simulink model "VehicleDynamics2011"  (Simulink 7.8)
settings: Solver=ode3  StartTime=0.0  StopTime=130  RelTol=1e-3
values from neighbouring files (symbols this model uses):
  b = 100    [parameters.m]
  L1 = 1.6    [parameters.m]
  m = 2000    [parameters.m]
undefined symbols (not defined in the file or in its folder): DiscIntNeverNeededParam
libraries: simulink x2
settings Model: Creator=jmapatel  LastModifiedBy=minzhe
settings OptimizationCC: InitFltsAndDblsToZero=on
settings DebuggingCC: SaveWithParameterizedLinksMsg=none  SignalResolutionControl=TryResolveAllWithWarning  MultiTaskDSMMsg=warning  MultiTaskCondExecSysMsg=none  FcnCallInpInsideContextMsg=Use local settings
settings CodeAppCC: CustomSymbolStrType=$N$R$M_T
settings GRTTargetCC: TargetFcnLib=ansi_tfl_tmw.mat  TargetFunctionLibrary=C89/C90 (ANSI)

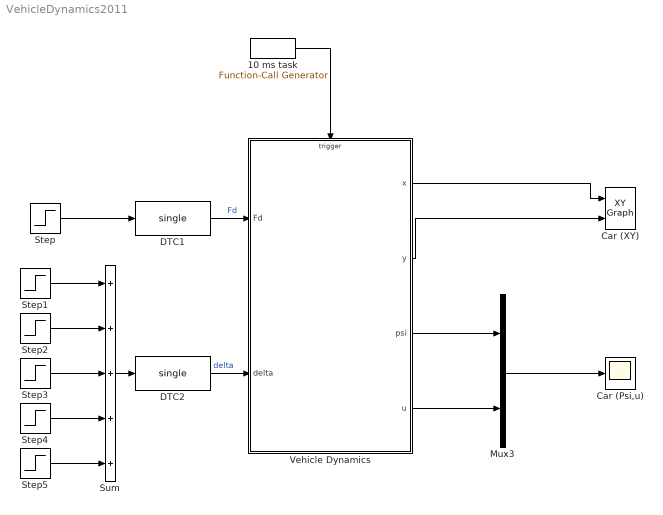
== system VehicleDynamics2011 ==
  10 ms task : simulink/Ports & Subsystems/Function-Call Generator  sample_time=0.01  numberOfIterations=1
  Car (Psi,u) : Scope
      settings: YMin=0  YMax=10  SaveName=ScopeData3
  Car (XY) : simulink/Sinks/XY Graph  xmin=-250  xmax=250  ymin=-250  ymax=250  st=-1
  DTC1 : DataTypeConversion  OutDataTypeStr=single
  DTC2 : DataTypeConversion  OutDataTypeStr=single
  Mux3 : Mux  Inputs=2
  Step : Step  After=1000
  Step1 : Step  Time=30  After=2*pi/180
  Step2 : Step  Time=50  After=-4*pi/180
  Step3 : Step  Time=70  After=5*pi/180
  Step4 : Step  Time=83  After=-3*pi/180
  Step5 : Step  Time=110  After=0.7*pi/180
  Sum : Sum  Inputs=+++++
  Vehicle Dynamics : Subsystem  TreatAsAtomicUnit=on
  wires:
  10 ms task/1 -> Vehicle Dynamics/Trigger
  Vehicle Dynamics/1(x) -> Car (XY)/1
  Vehicle Dynamics/2(y) -> Car (XY)/2
  Mux3/1 -> Car (Psi,u)/1
  Step/1 -> DTC1/1
  Sum/1 -> DTC2/1
  Step1/1 -> Sum/1
  Step2/1 -> Sum/2
  Step3/1 -> Sum/3
  Step4/1 -> Sum/4
  Step5/1 -> Sum/5
  DTC1/1 -> Vehicle Dynamics/1(Fd)  "Fd"
  DTC2/1 -> Vehicle Dynamics/2(delta)  "delta"
  Vehicle Dynamics/3(psi) -> Mux3/1
  Vehicle Dynamics/4(u) -> Mux3/2

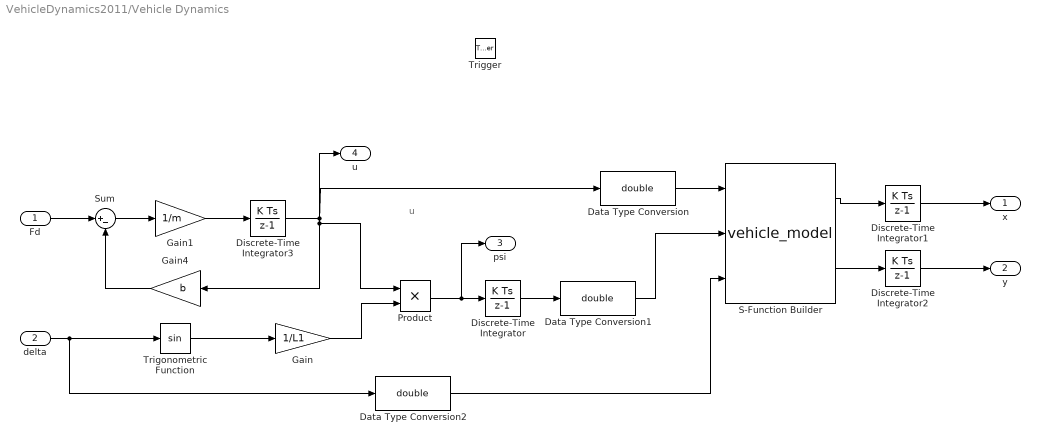
== system VehicleDynamics2011/Vehicle Dynamics ==
  note: u
  Fd : Inport
  delta : Inport  Port=2
  Trigger : TriggerPort  TriggerType=function-call
  Data Type Conversion : DataTypeConversion  OutDataTypeStr=double
  Data Type Conversion1 : DataTypeConversion  OutDataTypeStr=double
  Data Type Conversion2 : DataTypeConversion  OutDataTypeStr=double
  Discrete-Time Integrator : DiscreteIntegrator  SampleTime=-1  ICPrevOutput=DiscIntNeverNeededParam  ICPrevScaledInput=DiscIntNeverNeededParam
  Discrete-Time Integrator1 : DiscreteIntegrator  gainval=1  SampleTime=-1  ICPrevOutput=DiscIntNeverNeededParam  ICPrevScaledInput=DiscIntNeverNeededParam
  Discrete-Time Integrator2 : DiscreteIntegrator  gainval=1  SampleTime=-1  ICPrevOutput=DiscIntNeverNeededParam  ICPrevScaledInput=DiscIntNeverNeededParam
  Discrete-Time Integrator3 : DiscreteIntegrator  gainval=1  SampleTime=-1  ICPrevOutput=DiscIntNeverNeededParam  ICPrevScaledInput=DiscIntNeverNeededParam
  Gain : Gain  Gain=1/L1
  Gain1 : Gain  Gain=1/m
  Gain4 : Gain  Gain=b
  Product : Product
  S-Function Builder : S-Function  InitFcn=try, set_param(gcb,'FunctionName','vehicle_model'), end  FunctionName=vehicle_model  SFunctionModules=vehicle_model_wrapper  WizardData=DataTag0  EnableBusSupport=off  mask(S-Function Builder){}
      mask help: Simulink:masks:SFunctionBuilder_MD
      mask init:
      | val = [[.9  0.75 0.75 1 1 .9 .9 1]',[1 1 0.75 0.75 .9 .9 1 .9]'];try , sys = get_param(gcb,'SfunBuilderFcnName');if isempty(sys), sys = get_param(gcb,'FunctionName'); end,catch, sys = get_param(gcb,'FunctionName'); end
      settings: CopyFcn=set_param(gcbh,'LinkStatus','none')  PreSaveFcn=try, set_param(gcb,'FunctionName','vehicle_model'), end  OpenFcn=sfunctionwizard(gcbh)
      mask Display: plot(val(:,1),val(:,2)),disp(sys), port_label('input',1,'u'), port_label('input',2,'psi'), port_label('input',3,'delta'), port_label('output',1,'dotx'), port_label('output',2,'doty')
  Sum : Sum  Inputs=|+-
  Trigonometric Function : Trigonometry
  x : Outport
  y : Outport  Port=2
  psi : Outport  Port=3
  u : Outport  Port=4
  wires:
  delta/1 -> Data Type Conversion2/1, Trigonometric Function/1
  Trigonometric Function/1 -> Gain/1
  Gain/1 -> Product/2
  Product/1 -> psi/1, Discrete-Time Integrator/1
  Discrete-Time Integrator/1 -> Data Type Conversion1/1
  S-Function Builder/1 -> Discrete-Time Integrator1/1
  Discrete-Time Integrator1/1 -> x/1
  S-Function Builder/2 -> Discrete-Time Integrator2/1
  Discrete-Time Integrator2/1 -> y/1
  Sum/1 -> Gain1/1
  Gain1/1 -> Discrete-Time Integrator3/1
  Gain4/1 -> Sum/2
  Fd/1 -> Sum/1
  Discrete-Time Integrator3/1 -> Gain4/1, Product/1, Data Type Conversion/1, u/1
  Data Type Conversion/1 -> S-Function Builder/1
  Data Type Conversion1/1 -> S-Function Builder/2
  Data Type Conversion2/1 -> S-Function Builder/3
